simulink model "flightControlSystem"  (R2019b)
settings: Solver=ode3  StartTime=0  StopTime=TFinal  FixedStep=Ts  RelTol=1e-3  EnableMultiTasking=on
undefined symbols (not defined in the file): codertarget, Controller, DiscIntNeverNeededParam, Discrete, Estimator, g, init, Sensors, Time, Ts, Vehicle
libraries: simulink x35, vrlib x4, sharedtransform x3, ctrlSharedLib x2, sharedutil x1, parrotlib x1
(part 2 of 2)

== system flightControlSystem/Control System/Path Planning/Line Follower/Re-find track ==
  x_target : Inport  OutDataTypeStr=single
  y_target : Inport  Port=2  OutDataTypeStr=single
  x_cur : Inport  Port=3  OutDataTypeStr=single
  y_cur : Inport  Port=4  OutDataTypeStr=single
  MATLAB Function : MATLAB Function  TreatAsAtomicUnit=on
  Mux : Mux  Inputs=3
  Z_pos : Constant  Value=-1.1  OutDataTypeStr=single
  target_coordinates : Outport  OutDataTypeStr=single
  wires:
  Mux/1 -> target_coordinates/1
  Z_pos/1 -> Mux/3
  y_target/1 -> MATLAB Function/3(y_target)
  y_cur/1 -> MATLAB Function/4(y_cur)
  x_target/1 -> MATLAB Function/1(x_target)
  x_cur/1 -> MATLAB Function/2(x_cur)
  MATLAB Function/2(y) -> Mux/2
  MATLAB Function/1(x) -> Mux/1

== system flightControlSystem/Control System/State Estimator/Complementary Filter/If Action Subsystem ==
  rpy : Inport
  accel : Inport  Port=2
  Action Port : ActionPort  ActionPortLabel=if(u1 > 0)
  Demux : Demux  Outputs=3
  Demux1 : Demux  Outputs=3
  Divide : Product  Inputs=*/
  Gain : Gain  Gain=1-Estimator.gyroAngleUpdateAccWeight
  Gain1 : Gain  Gain=Estimator.gyroAngleUpdateAccWeight
  Gain2 : Gain  Gain=1/g
  Gain3 : Gain  Gain=Estimator.gyroAngleUpdateAccWeight
  Gain4 : Gain  Gain=1-Estimator.gyroAngleUpdateAccWeight
  Mux : Mux  Inputs=2
  Sum : Sum  Inputs=|++
  Sum1 : Sum  Inputs=|++
  Terminator1 : Terminator
  Trigonometric Function : Trigonometry  Operator=atan
  Trigonometric Function1 : Trigonometry  Operator=asin
  pitch,roll : Outport  VectorParamsAs1DForOutWhenUnconnected=off
  wires:
  accel/1 -> Demux/1
  Demux/2 -> Divide/1
  Demux/3 -> Divide/2
  Divide/1 -> Trigonometric Function/1
  Gain/1 -> Sum/1
  Trigonometric Function/1 -> Gain1/1
  Mux/1 -> pitch,roll/1
  Gain2/1 -> Trigonometric Function1/1
  Trigonometric Function1/1 -> Gain3/1
  Gain4/1 -> Sum1/1
  Gain3/1 -> Sum1/2
  Sum1/1 -> Mux/1
  Sum/1 -> Mux/2
  rpy/1 -> Demux1/1
  Demux1/1 -> Gain/1
  Demux1/2 -> Gain4/1
  Demux/1 -> Gain2/1
  Demux1/3 -> Terminator1/1
  Gain1/1 -> Sum/2

== system flightControlSystem/Control System/State Estimator/Complementary Filter/If Action Subsystem2 ==
  prin : Inport
  Action Port : ActionPort  ActionPortLabel=else
  prout : Outport  VectorParamsAs1DForOutWhenUnconnected=off
  wires:
  prin/1 -> prout/1

== system flightControlSystem/Control System/State Estimator/Complementary Filter/Wbe ==
  rpy : Inport  OutDataTypeStr=single
  Constant : Constant  Value=single(0)
  Create 3x3 Matrix : sharedutil/Create 3x3 Matrix  aMode=aMode
  Divide : Product  Inputs=*/
  Gain : Gain  Gain=-1
  Product{1..4} (4 alike) : Product
  Selector : Selector  InputPortWidth=3  IndexOptions=Index vector (dialog)  Indices=[1]  OutputSizes=1
  Selector1 : Selector  InputPortWidth=3  IndexOptions=Index vector (dialog)  Indices=[1]  OutputSizes=1
  Selector2 : Selector  InputPortWidth=3  IndexOptions=Index vector (dialog)  Indices=[2]  OutputSizes=1
  Selector3 : Selector  InputPortWidth=3  IndexOptions=Index vector (dialog)  Indices=[2]  OutputSizes=1
  Trigonometric Function : Trigonometry  Operator=sincos
  Wbe : Outport  VectorParamsAs1DForOutWhenUnconnected=off
  wires:
  Create 3x3 Matrix/1 -> Divide/1
  Product3/1 -> Create 3x3 Matrix/8
  Trigonometric Function/2 -> Selector1/1, Selector2/1
  Selector3/1 -> Product4/2, Product3/2
  Selector1/1 -> Product4/1, Product1/1, Create 3x3 Matrix/3
  Trigonometric Function/1 -> Selector3/1, Selector/1
  Product1/1 -> Create 3x3 Matrix/5
  Product2/1 -> Create 3x3 Matrix/6
  Selector2/1 -> Divide/2, Create 3x3 Matrix/7, Product2/1, Product1/2
  Gain/1 -> Product2/2
  Product4/1 -> Create 3x3 Matrix/9
  Constant/1 -> Create 3x3 Matrix/4, Create 3x3 Matrix/1
  Divide/1 -> Wbe/1
  rpy/1 -> Trigonometric Function/1
  Selector/1 -> Product3/1, Gain/1, Create 3x3 Matrix/2

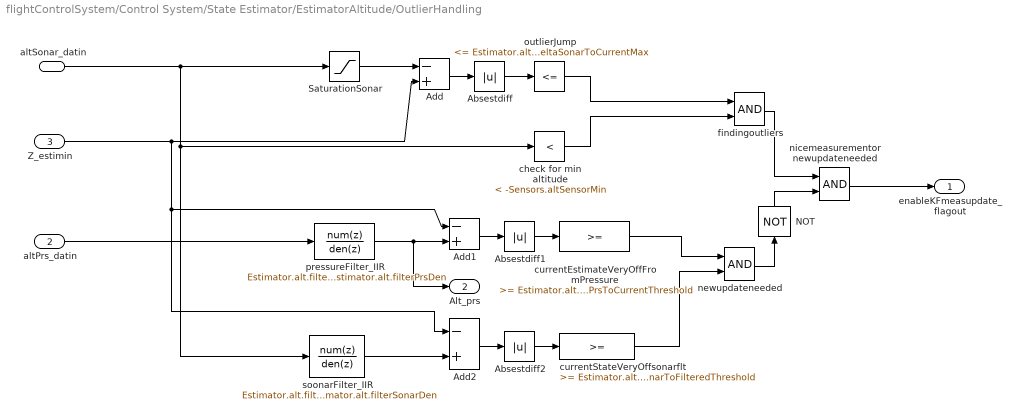
== system flightControlSystem/Control System/State Estimator/EstimatorAltitude/OutlierHandling ==
  altSonar_datin : Inport
  altPrs_datin : Inport  Port=2
  Z_estimin : Inport  Port=3
  Absestdiff : Abs
  Absestdiff1 : Abs
  Absestdiff2 : Abs
  Add : Sum  Inputs=-+
  Add1 : Sum  Inputs=-+
  Add2 : Sum  Inputs=-+
  NOT : Logic  Operator=NOT  IconShape=distinctive  AllPortsSameDT=off  OutDataTypeStr=boolean
  SaturationSonar : Saturate  UpperLimit=-Sensors.altSensorMin  LowerLimit=-inf
  check for min altitude : simulink/Logic and Bit Operations/Compare To Constant  relop=<  const=-Sensors.altSensorMin  OutDataTypeStr=boolean
  currentEstimateVeryOffFromPressure : simulink/Logic and Bit Operations/Compare To Constant  relop=>=  const=Estimator.alt.deltaPrsToCurrentThreshold  OutDataTypeStr=boolean
  currentStateVeryOffsonarflt : simulink/Logic and Bit Operations/Compare To Constant  relop=>=  const=Estimator.alt.deltaSonarToFilteredThreshold  OutDataTypeStr=boolean
  findingoutliers : Logic  AllPortsSameDT=off  OutDataTypeStr=boolean
  newupdateneeded : Logic  AllPortsSameDT=off  OutDataTypeStr=boolean
  nicemeasurementor newupdateneeded : Logic  AllPortsSameDT=off  OutDataTypeStr=boolean
  outlierJump : simulink/Logic and Bit Operations/Compare To Constant  relop=<=  const=Estimator.alt.deltaSonarToCurrentMax  OutDataTypeStr=boolean
  pressureFilter_IIR : DiscreteFilter  Numerator=Estimator.alt.filterPrsNum  Denominator=Estimator.alt.filterPrsDen
  soonarFilter_IIR : DiscreteFilter  Numerator=Estimator.alt.filterSonarNum  Denominator=Estimator.alt.filterSonarDen
  enableKFmeasupdate_flagout : Outport  VectorParamsAs1DForOutWhenUnconnected=off
  Alt_prs : Outport  Port=2  VectorParamsAs1DForOutWhenUnconnected=off
  wires:
  Add1/1 -> Absestdiff1/1
  nicemeasurementor newupdateneeded/1 -> enableKFmeasupdate_flagout/1
  findingoutliers/1 -> nicemeasurementor newupdateneeded/1
  check for min altitude/1 -> findingoutliers/2
  outlierJump/1 -> findingoutliers/1
  SaturationSonar/1 -> Add/1
  Absestdiff/1 -> outlierJump/1
  Add/1 -> Absestdiff/1
  newupdateneeded/1 -> NOT/1
  Absestdiff2/1 -> currentStateVeryOffsonarflt/1
  altSonar_datin/1 -> SaturationSonar/1, soonarFilter_IIR/1, check for min altitude/1
  currentEstimateVeryOffFromPressure/1 -> newupdateneeded/1
  Z_estimin/1 -> Add1/1, Add2/1, Add/2
  Add2/1 -> Absestdiff2/1
  currentStateVeryOffsonarflt/1 -> newupdateneeded/2
  pressureFilter_IIR/1 -> Alt_prs/1, Add1/2
  altPrs_datin/1 -> pressureFilter_IIR/1
  soonarFilter_IIR/1 -> Add2/2
  Absestdiff1/1 -> currentEstimateVeryOffFromPressure/1
  NOT/1 -> nicemeasurementor newupdateneeded/2

== system flightControlSystem/Control System/State Estimator/EstimatorXYPosition/EstimatorVelocity ==
  opticalFlow_datin : Inport
  Z_estimin : Inport  Port=2  SampleTime=Ts
  sensorIMU_datin : Inport  Port=3
  orient_estimin : Inport  Port=4
  " " : Product  Inputs=**
  AccelerationHandling : Subsystem
  Compare To Constant : simulink/Logic and Bit Operations/Compare To Constant  relop=<  const=200*4  OutDataTypeStr=boolean
  Counter Free-Running : simulink/Sources/Counter Free-Running  NumBits=32  tsamp=-1
  DataHandling : Subsystem
  Delay : Delay  DelayLength=1  InitialCondition=0
  Gain : Gain  Gain=-1
  KalmanFilter_dxdy : ctrlSharedLib/Kalman Filter  TimeDomain=Discrete-Time  UseCurrentEstimator=on  ModelSource=Individual A, B, C, D matrices  ModelSourceVariable=ss(0.95,1,1,0,1)  A=eye(2)  B=Ts*eye(2)  C=eye(2)  D=0  NumberOfStates=1  NumberOfInputs=1  NumberOfOutputs=1  InitialEstimateSource=Dialog  X0=0  P0=10  UseK=off  UseGH=on  NumberOfProcessNoiseInputs=1  G=Estimator.pos.kfVelo.G  TimeInvariantG=on  H=Estimator.pos.kfVelo.H  TimeInvariantH=on  Q=Estimator.pos.kfVelo.Q  TimeInvariantQ=on  R=Estimator.pos.kfVelo.R  TimeInvariantR=on  N=Estimator.pos.kfVelo.N  TimeInvariantN=on  AddInputPort=on  AddEnablePort=on  OutputEstimatedY=off  OutputP=off  Ts=-1
      settings: SourceProductBaseCode=CT
  Select dxy : Selector  InputPortWidth=3  IndexOptions=Index vector (dialog)  Indices=[1 2]  OutputSizes=1
  Switch : Switch  Criteria=u2 > Threshold
  Z_estimin1 : InportShadow  Port=2  SampleTime=Ts
  opticalFlowErrorCorrect : Gain  Gain=1.15
  dxy_estimout : Outport  VectorParamsAs1DForOutWhenUnconnected=off
  wires:
  Delay/1 -> DataHandling/5(dxyOF_datin)
  Z_estimin/1 -> DataHandling/1(Z_estimin), AccelerationHandling/4(Z_estimin)
  KalmanFilter_dxdy/1 -> dxy_estimout/1, Delay/1
  sensorIMU_datin/1 -> AccelerationHandling/2(sensorIMU_datin), DataHandling/3(sensorIMU_datin)
  orient_estimin/1 -> AccelerationHandling/3(orient_estimin), DataHandling/2(orient_estimin)
  Select dxy/1 -> KalmanFilter_dxdy/2, AccelerationHandling/1(dxy_estimin), DataHandling/4(dxy_estimin)
  AccelerationHandling/1(acceleration_world) -> KalmanFilter_dxdy/1
  DataHandling/1(enable_flag) -> KalmanFilter_dxdy/3
  Switch/1 -> Select dxy/1
  " "/1 -> opticalFlowErrorCorrect/1
  Gain/1 -> " "/2
  opticalFlowErrorCorrect/1 -> Switch/3
  Compare To Constant/1 -> Switch/2
  opticalFlow_datin/1 -> " "/1, Switch/1
  Z_estimin1/1 -> Gain/1
  Counter Free-Running/1 -> Compare To Constant/1

== system flightControlSystem/Control System/State Estimator/EstimatorXYPosition/EstimatorXYPosition ==
  note: Switching from orientationControl to Position
      | control reset the current world position estimate
      | (happens when using no markers)
  dxy_estimin : Inport
  orient_estimin : Inport  Port=2  SampleTime=Ts
  controlModePosVSOrient_flagin : Inport  Port=3
  dz_estimin : Inport  Port=4
  Math Function : Math  Operator=transpose  SaturateOnIntegerOverflow=on
  Mux2 : Mux  Inputs=2
  Product : Product  Multiplication=Matrix(*)
  Rotation Angles to Direction Cosine Matrix : sharedtransform/Rotation Angles to Direction Cosine Matrix  rotationOrder=ZYX  aMode=aMode
      settings: SourceProductBaseCode=AE
  SelectdXY : Selector  InputPortWidth=3  IndexOptions=Index vector (dialog)  Indices=[1 2]  OutputSizes=1
  SimplyIntegrateVelocity : DiscreteIntegrator  ExternalReset=rising  SampleTime=Ts  ICPrevOutput=DiscIntNeverNeededParam  ICPrevScaledInput=DiscIntNeverNeededParam
  XY_estimout : Outport  VectorParamsAs1DForOutWhenUnconnected=off
  wires:
  controlModePosVSOrient_flagin/1 -> SimplyIntegrateVelocity/2
  Product/1 -> SelectdXY/1
  Mux2/1 -> Product/2
  dz_estimin/1 -> Mux2/2
  SimplyIntegrateVelocity/1 -> XY_estimout/1
  dxy_estimin/1 -> Mux2/1
  orient_estimin/1 -> Rotation Angles to Direction Cosine Matrix/1
  Rotation Angles to Direction Cosine Matrix/1 -> Math Function/1
  SelectdXY/1 -> SimplyIntegrateVelocity/1
  Math Function/1 -> Product/1

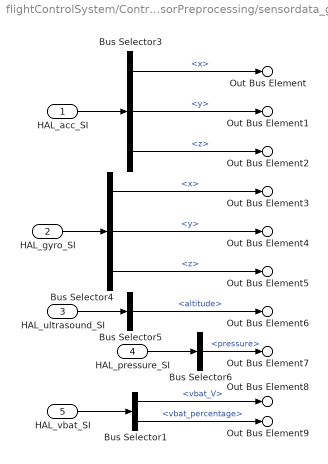
== system flightControlSystem/Control System/State Estimator/SensorPreprocessing/sensordata_group ==
  HAL_acc_SI : Inport  OutDataTypeStr=Bus: HAL_acc_SI_t
  HAL_gyro_SI : Inport  Port=2  OutDataTypeStr=Bus: HAL_gyro_SI_t
  HAL_ultrasound_SI : Inport  Port=3  OutDataTypeStr=Bus: HAL_ultrasound_SI_t
  HAL_pressure_SI : Inport  Port=4  OutDataTypeStr=Bus: HAL_pressure_SI_t
  HAL_vbat_SI : Inport  Port=5  OutDataTypeStr=Bus: HAL_vbat_SI_t
  Bus Selector1 : BusSelector  OutputSignals=vbat_V,vbat_percentage
  Bus Selector3 : BusSelector  OutputSignals=x,y,z
  Bus Selector4 : BusSelector  OutputSignals=x,y,z
  Bus Selector5 : BusSelector  OutputSignals=altitude
  Bus Selector6 : BusSelector  OutputSignals=pressure
  Out Bus Element : Outport  VectorParamsAs1DForOutWhenUnconnected=off  PortName=sensordata_datin  Element=ddx
  Out Bus Element1 : Outport  VectorParamsAs1DForOutWhenUnconnected=off  PortName=sensordata_datin  Element=ddy
  Out Bus Element2 : Outport  VectorParamsAs1DForOutWhenUnconnected=off  PortName=sensordata_datin  Element=ddz
  Out Bus Element3 : Outport  VectorParamsAs1DForOutWhenUnconnected=off  PortName=sensordata_datin  Element=p
  Out Bus Element4 : Outport  VectorParamsAs1DForOutWhenUnconnected=off  PortName=sensordata_datin  Element=q
  Out Bus Element5 : Outport  VectorParamsAs1DForOutWhenUnconnected=off  PortName=sensordata_datin  Element=r
  Out Bus Element6 : Outport  VectorParamsAs1DForOutWhenUnconnected=off  PortName=sensordata_datin  Element=altitude_sonar
  Out Bus Element7 : Outport  VectorParamsAs1DForOutWhenUnconnected=off  PortName=sensordata_datin  Element=prs
  Out Bus Element8 : Outport  VectorParamsAs1DForOutWhenUnconnected=off  PortName=sensordata_datin  Element=vbat_V
  Out Bus Element9 : Outport  VectorParamsAs1DForOutWhenUnconnected=off  PortName=sensordata_datin  Element=vbat_percentage
  wires:
  HAL_gyro_SI/1 -> Bus Selector4/1
  HAL_acc_SI/1 -> Bus Selector3/1
  HAL_pressure_SI/1 -> Bus Selector6/1
  HAL_ultrasound_SI/1 -> Bus Selector5/1
  Bus Selector4/1 -> Out Bus Element3/1  "<x>"
  Bus Selector3/3 -> Out Bus Element2/1  "<z>"
  Bus Selector4/3 -> Out Bus Element5/1  "<z>"
  Bus Selector5/1 -> Out Bus Element6/1  "<altitude>"
  Bus Selector6/1 -> Out Bus Element7/1  "<pressure>"
  Bus Selector4/2 -> Out Bus Element4/1  "<y>"
  Bus Selector3/1 -> Out Bus Element/1  "<x>"
  Bus Selector3/2 -> Out Bus Element1/1  "<y>"
  Bus Selector1/1 -> Out Bus Element8/1  "<vbat_V>"
  HAL_vbat_SI/1 -> Bus Selector1/1
  Bus Selector1/2 -> Out Bus Element9/1  "<vbat_percentage>"

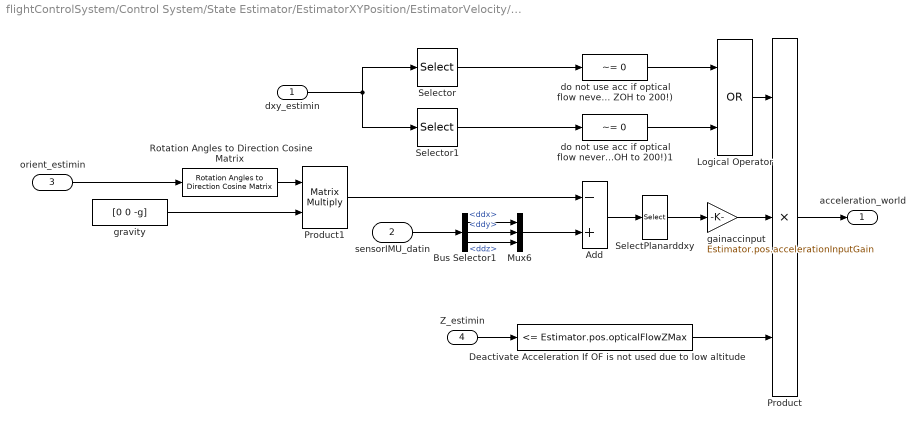
== system flightControlSystem/Control System/State Estimator/EstimatorXYPosition/EstimatorVelocity/AccelerationHandling ==
  dxy_estimin : Inport
  sensorIMU_datin : Inport  Port=2
  orient_estimin : Inport  Port=3
  Z_estimin : Inport  Port=4
  Add : Sum  Inputs=-+
  Bus Selector1 : BusSelector  OutputSignals=ddx,ddy,ddz
  Deactivate Acceleration If OF is not used due to low altitude : simulink/Logic and Bit Operations/Compare To Constant  relop=<=  const=Estimator.pos.opticalFlowZMax  OutDataTypeStr=boolean
  Logical Operator : Logic  Operator=OR  AllPortsSameDT=off  OutDataTypeStr=boolean
  Mux6 : Mux  Inputs=3
  Product : Product  Inputs=3
  Product1 : Product  Multiplication=Matrix(*)
  Rotation Angles to Direction Cosine Matrix : sharedtransform/Rotation Angles to Direction Cosine Matrix  rotationOrder=ZYX  aMode=aMode
      settings: SourceProductBaseCode=AE
  SelectPlanarddxy : Selector  InputPortWidth=3  IndexOptions=Index vector (dialog)  Indices=[1 2]  OutputSizes=1
  Selector : Selector  InputPortWidth=2  IndexOptions=Index vector (dialog)  Indices=1  OutputSizes=1
  Selector1 : Selector  InputPortWidth=2  IndexOptions=Index vector (dialog)  Indices=2  OutputSizes=1
  do not use acc if optical flow never available (Note OF@60Hz but ZOH to 200!) : simulink/Logic and Bit Operations/Compare To Constant  relop=~=  const=0  OutDataTypeStr=boolean
  do not use acc if optical flow never available (Note OF@60Hz but ZOH to 200!)1 : simulink/Logic and Bit Operations/Compare To Constant  relop=~=  const=0  OutDataTypeStr=boolean
  gainaccinput : Gain  Gain=Estimator.pos.accelerationInputGain  OutDataTypeStr=single
  gravity : Constant  Value=[0 0 -g]
  acceleration_world : Outport  OutDataTypeStr=single  VectorParamsAs1DForOutWhenUnconnected=off
  wires:
  do not use acc if optical flow never available (Note OF@60Hz but ZOH to 200!)1/1 -> Logical Operator/2
  do not use acc if optical flow never available (Note OF@60Hz but ZOH to 200!)/1 -> Logical Operator/1
  Logical Operator/1 -> Product/1
  Selector1/1 -> do not use acc if optical flow never available (Note OF@60Hz but ZOH to 200!)1/1
  Selector/1 -> do not use acc if optical flow never available (Note OF@60Hz but ZOH to 200!)/1
  dxy_estimin/1 -> Selector1/1, Selector/1
  Product/1 -> acceleration_world/1
  Deactivate Acceleration If OF is not used due to low altitude/1 -> Product/3
  Z_estimin/1 -> Deactivate Acceleration If OF is not used due to low altitude/1
  Add/1 -> SelectPlanarddxy/1
  Product1/1 -> Add/1
  gravity/1 -> Product1/2
  gainaccinput/1 -> Product/2
  SelectPlanarddxy/1 -> gainaccinput/1
  Bus Selector1/3 -> Mux6/3  "<ddz>"
  Bus Selector1/1 -> Mux6/1  "<ddx>"
  sensorIMU_datin/1 -> Bus Selector1/1
  Mux6/1 -> Add/2
  Bus Selector1/2 -> Mux6/2  "<ddy>"
  orient_estimin/1 -> Rotation Angles to Direction Cosine Matrix/1
  Rotation Angles to Direction Cosine Matrix/1 -> Product1/1

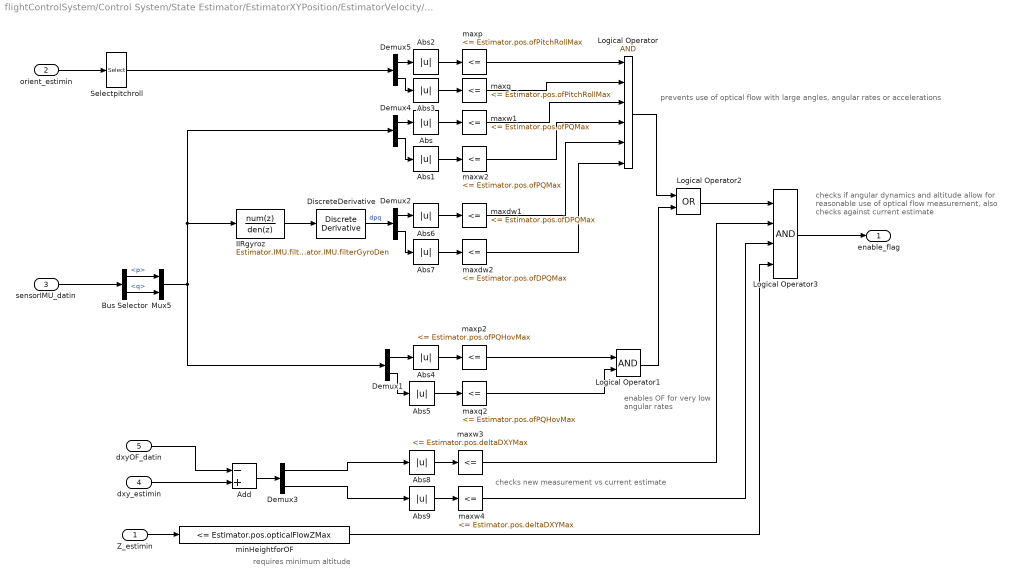
== system flightControlSystem/Control System/State Estimator/EstimatorXYPosition/EstimatorVelocity/DataHandling ==
  note: prevents use of optical flow with large angles, angular rates or accelerations
  note: enables OF for very
      | low angular rates
  note: checks if angular dynamics and altitude allow for
      | reasonable use of optical flow measurement,
      | also checks against current estimate
  note: checks new measurement vs current estimate
  note: requires minimum altitude
  Z_estimin : Inport
  orient_estimin : Inport  Port=2
  sensorIMU_datin : Inport  Port=3
  dxy_estimin : Inport  Port=4
  dxyOF_datin : Inport  Port=5
  Abs{,1..9} (10 alike) : Abs
  Add : Sum  Inputs=-+
  Bus Selector : BusSelector  OutputSignals=p,q
  Demux{1..5} (5 alike) : Demux  Outputs=2
  DiscreteDerivative : simulink/Discrete/Discrete Derivative  gainval=1.0  ICPrevScaledInput=0.0  OutMin=[]  OutMax=[]  OutDataType=fixdt(1, 16)  OutScaling=2^-10  DoSatur=off
  IIRgyroz : DiscreteFilter  Numerator=Estimator.IMU.filterGyroNum  Denominator=Estimator.IMU.filterGyroDen
  Logical Operator : Logic  Inputs=6  AllPortsSameDT=off  OutDataTypeStr=boolean
  Logical Operator1 : Logic  AllPortsSameDT=off  OutDataTypeStr=boolean
  Logical Operator2 : Logic  Operator=OR  AllPortsSameDT=off  OutDataTypeStr=boolean
  Logical Operator3 : Logic  Inputs=4  AllPortsSameDT=off  OutDataTypeStr=boolean
  Mux5 : Mux  Inputs=2
  Selectpitchroll : Selector  InputPortWidth=3  IndexOptions=Index vector (dialog)  Indices=[2 3]  OutputSizes=1
  maxdw1 : simulink/Logic and Bit Operations/Compare To Constant  relop=<=  const=Estimator.pos.ofDPQMax  OutDataTypeStr=boolean
  maxdw2 : simulink/Logic and Bit Operations/Compare To Constant  relop=<=  const=Estimator.pos.ofDPQMax  OutDataTypeStr=boolean
  maxp : simulink/Logic and Bit Operations/Compare To Constant  relop=<=  const=Estimator.pos.ofPitchRollMax  OutDataTypeStr=boolean
  maxp2 : simulink/Logic and Bit Operations/Compare To Constant  relop=<=  const=Estimator.pos.ofPQHovMax  OutDataTypeStr=boolean
  maxq : simulink/Logic and Bit Operations/Compare To Constant  relop=<=  const=Estimator.pos.ofPitchRollMax  OutDataTypeStr=boolean
  maxq2 : simulink/Logic and Bit Operations/Compare To Constant  relop=<=  const=Estimator.pos.ofPQHovMax  OutDataTypeStr=boolean
  maxw1 : simulink/Logic and Bit Operations/Compare To Constant  relop=<=  const=Estimator.pos.ofPQMax  OutDataTypeStr=boolean
  maxw2 : simulink/Logic and Bit Operations/Compare To Constant  relop=<=  const=Estimator.pos.ofPQMax  OutDataTypeStr=boolean
  maxw3 : simulink/Logic and Bit Operations/Compare To Constant  relop=<=  const=Estimator.pos.deltaDXYMax  OutDataTypeStr=boolean
  maxw4 : simulink/Logic and Bit Operations/Compare To Constant  relop=<=  const=Estimator.pos.deltaDXYMax  OutDataTypeStr=boolean
  minHeightforOF : simulink/Logic and Bit Operations/Compare To Constant  relop=<=  const=Estimator.pos.opticalFlowZMax  OutDataTypeStr=boolean
  enable_flag : Outport  VectorParamsAs1DForOutWhenUnconnected=off
  wires:
  minHeightforOF/1 -> Logical Operator3/4
  IIRgyroz/1 -> DiscreteDerivative/1
  Mux5/1 -> Demux1/1, IIRgyroz/1, Demux4/1
  maxw4/1 -> Logical Operator3/3
  maxw3/1 -> Logical Operator3/2
  dxyOF_datin/1 -> Add/1
  Demux3/2 -> Abs9/1
  Demux3/1 -> Abs8/1
  dxy_estimin/1 -> Add/2
  Add/1 -> Demux3/1
  Abs9/1 -> maxw4/1
  Abs8/1 -> maxw3/1
  Logical Operator2/1 -> Logical Operator3/1
  Logical Operator3/1 -> enable_flag/1
  DiscreteDerivative/1 -> Demux2/1  "dpq"
  Demux2/2 -> Abs7/1
  Demux2/1 -> Abs6/1
  Abs7/1 -> maxdw2/1
  Abs6/1 -> maxdw1/1
  Logical Operator1/1 -> Logical Operator2/2
  Demux1/2 -> Abs5/1
  Demux1/1 -> Abs4/1
  Abs5/1 -> maxq2/1
  Abs4/1 -> maxp2/1
  Abs3/1 -> maxq/1
  Abs2/1 -> maxp/1
  Demux4/2 -> Abs1/1
  Demux4/1 -> Abs/1
  Abs1/1 -> maxw2/1
  Abs/1 -> maxw1/1
  Z_estimin/1 -> minHeightforOF/1
  Logical Operator/1 -> Logical Operator2/1
  maxw1/1 -> Logical Operator/3
  Bus Selector/1 -> Mux5/1  "<p>"
  Selectpitchroll/1 -> Demux5/1
  sensorIMU_datin/1 -> Bus Selector/1
  maxq2/1 -> Logical Operator1/2
  Bus Selector/2 -> Mux5/2  "<q>"
  maxp/1 -> Logical Operator/1
  maxw2/1 -> Logical Operator/4
  orient_estimin/1 -> Selectpitchroll/1
  maxdw1/1 -> Logical Operator/5
  maxdw2/1 -> Logical Operator/6
  maxq/1 -> Logical Operator/2
  Demux5/1 -> Abs2/1
  Demux5/2 -> Abs3/1
  maxp2/1 -> Logical Operator1/1

== matlab function flightControlSystem/Image Processing System/Circle Finder ==
  data: BW input; circleFound output; coordinates output
function [circleFound, coordinates] = FindTheCircle(BW)

red = 0;

circleFound = false;
coordinates = [0,0];
row = 120;
col = 160;

%%%%NEEDS FOCUS
diameter = 37;
margin = 1; 

%stepsize = 1; %e.g. could change to 2 to check every 2nd column
for i = 1:1:col %traverse columns in BW image
    red_px_count = 0; %count of consecutive red pixels in a column - is updated as we traverse columns
    for j = 1:1:(row - 1) %traverse rows in column - not to last row element
        %Adjusting red_px_count 
        if (BW(j,i) == red) %i.e. if pixel is red
            red_px_count = red_px_count + 1;
        else 
            red_px_count = 0;
        end
        
        if ( (red_px_count <= diameter + margin) && (red_px_count >= diameter - margin) && (BW(j+1,i) ~= red))
            %centre row is around/at (j - (red_px_count-1)/2) depending on
            %whether result is a decimal or integer
            row_pos = (j - (red_px_count-1)/2);
            if( horizontal_test(floor(row_pos),i,BW) == true )
                circleFound = true;
                coordinates = [i,floor(row_pos)]; %returning col,row format as thats what is currently expected at path planning
                break;
            elseif (horizontal_test(ceil(row_pos),i,BW) == true )
                circleFound = true;
                coordinates = [i, ceil(row_pos)]; %col, row format
                break;
            end
        end
    end
end

function circleFound = horizontal_test(row,col,BW)

red = 0;

num_col = 160;
circleFound = false;

diameter = 37;
diameter_margin = 1;

centre_margin = 1;
red_px_count = 0; %count of consecutive red pixels in a column - is updated as we traverse columns

for i = 1:1:(num_col-1) %traverse columns in BW image
        %Adjusting red_px_count
        if (BW(row,i) == red) %i.e. if pixel is red
            red_px_count = red_px_count + 1;
        else
            red_px_count = 0;
        end
        %Checking if red_px_count = ~ diameter of circle
        if ( (red_px_count <= diameter + diameter_margin) && (red_px_count >= diameter - diameter_margin) && BW(row,i+1) ~= red )
            col_no = i - (red_px_count - 1)/2;
            if ( col_no <= col + centre_margin && col_no >= col - centre_margin )
                circleFound = true;
                break;
            end
        end
end

== matlab function flightControlSystem/Image Processing System/MATLAB Function1 ==
  data: r input; r1 output; g input; b input; av_points input; g1 output; b1 output
%FUNCTION DESCRIPTION

% the values for r1,g1,b1 which we pass out are the same as r,g,b inputs
% except r1,g1,b1 values are changed to highlight: 
%
% - origin/centre of image
% 
% - gridlines used in 'Waypoint Finder' block
% 
% - 4 average points along 4 gridlines used to calculate unit vectors in
%  'Waypoint Finder' block

function [r1,g1,b1] = fcn(r,g,b,av_points)
% setting values for r1,g1,b1 equal to r,g,b inputs
r1=r;
g1=g;
b1=b;

% highlighting origin (centre of image) black (black's r,g,b value is 1,1,1)
r1(60,80) = 1;
g1(60,80) = 1;
b1(60,80) = 1;


% highlighting gridlines used in 'Waypoint Finder' block black
% (black's r,g,b value is 1,1,1)
% gridline 1
r1(40,:) = 1;
g1(40,:) = 1;
b1(40,:) = 1;

% gridline 2
r1(80,:) = 1;
g1(80,:) = 1;
b1(80,:) = 1;

% gridline 3
r1(:,60) = 1;
g1(:,60) = 1;
b1(:,60) = 1;

% gridline 4
r1(:,100) = 1;
g1(:,100) = 1;
b1(:,100) = 1;

% highlighting av_points white if valid points are received hence isnan
%(white's r,g,b value is 255,255,255)

% point 1
if ~isnan(av_points(1:2))
r1(av_points(1),av_points(2)) = 255;
g1(av_points(1),av_points(2)) = 255;
b1(av_points(1),av_points(2)) = 255;
end

% point 2
if ~isnan(av_points(3:4))
r1(av_points(3),av_points(4)) = 255;
g1(av_points(3),av_points(4)) = 255;
b1(av_points(3),av_points(4)) = 255;
end

% point 3
if ~isnan(av_points(5:6))
r1(av_points(5),av_points(6)) = 255;
g1(av_points(5),av_points(6)) = 255;
b1(av_points(5),av_points(6)) = 255;
end

% point 4
if ~isnan(av_points(7:8))
r1(av_points(7),av_points(8)) = 255;
g1(av_points(7),av_points(8)) = 255;
b1(av_points(7),av_points(8)) = 255;
end

== matlab function flightControlSystem/Image Processing System/rgb to boolean ==
  data: r input; BW output; g input; b input
function BW = fcn(r, g, b)
%Threshold values for r,g,b components
Th_r = 190;
Th_g = 90;
Th_b = 90;

BW = ~( r > Th_r & g < Th_g & b < Th_b);

== matlab function flightControlSystem/Control System/Path Planning/Go to centre/Coord to Vector ==
  data: coord input; x_vec output; y_vec output; z_vec output; over_centre output; yaw input; pitch input; roll input
function [x_vec, y_vec, z_vec, over_centre] = fcn(coord,yaw,pitch,roll)
%This function will take the coordinates of the target circle with the top
%left pixel as the origin and convert it to a vector with the origin as the
%centre of the image.
%It then tells the drone to land at it's centre

%Input: coord, coordinates of target circle
%Output: vec2target, vector to center pointing from center of image
%       x_vec, x component of vector to fly to
%       y_vec, same as for x_vec
%       z_vec, same as for x_vec
%       over_centre, flag for when over circle
    %radius = 19;
    threshold = 10;
    %Convert coordinate space to origin at centre
    coord = coord - [80, 60]; %Pixel positions with centre as origin
    vec2target = coord.*[1, -1];
    
    nrm = norm(vec2target);
    x_vec = vec2target(2)/nrm;
    y_vec = vec2target(1)/nrm;
    z_vec = -1.1;
    over_centre = false;
    
    %Tell drone to land if above the circle
    if ( nrm < threshold & yaw < 0.0001 & pitch < 0.0001 & roll < 0.0001 )
        x_vec = 0;
        y_vec = 0;
        over_centre = true;
    end

== stateflow chart flightControlSystem/Control System/Path Planning/Line Follower/State Machine ==
  state Lost
    entry:
    mode = 1;
    last_valid_vec = [(xp - xp_min1) (yp - yp_min1)];
    x_target = (xp+xp_min1)/2;
    y_target = (yp+yp_min1)/2;
  state NormalOp
    entry:
    mode = 0;
    during:
    last_valid_vec = [(xcur - xcur_minus1) (ycur - ycur_minus1)];
  (default) -> NormalOp
  NormalOp -> Lost : [lost]
  Lost -> NormalOp : [~lost & abs(xcur-x_target) < closeness_margin & abs(ycur-y_target) < closeness_margin]
  data: lost input; mode output; xcur input; xcur_minus1 input; ycur input; ycur_minus1 input; last_valid_vec output; closeness_margin constant double =0.005; x_target output single; y_target output single; xp input; xp_min1 input; yp input; yp_min1 input

== matlab function flightControlSystem/Control System/Path Planning/Line Follower/MATLAB Function ==
  data: vecs input; lost output
function lost  = fcn(vecs)
vecs_nan = isnan(vecs);
if( (vecs_nan(1) || vecs_nan(2)) && (vecs_nan(3) || vecs_nan(4)) && (vecs_nan(5) || vecs_nan(6)) && (vecs_nan(7) || vecs_nan(8)) )
    lost = true;
else
    lost = false;
end

== matlab function flightControlSystem/Control System/Path Planning/Line Follower/Normal Operation/Best Path ==
  data: vecs input; x_best output; last_travelled_vec input; y_best output
%vecs = [y1, x1, y2, x2, y3, x3, y4, x4]
%-> array containing up to 4 valid unit vectors
 
%We will choose the unit vector from vecs which is most similar to the 
%unit vector we travelled (in the direction of) in the previous time step
 
%i.e. We choose the vector from vecs which gives the largest value 
%from this eq.
%(x_p + vecs[xi])^2 + (y_p + vecs[yi]))^2 
 
%e.g. if one vector told us to go back relative to direction we were 
%just travelling, it's x and y components would cancel with the x and 
%y components of the vector we last travelled through and we would discount
%it as a valid vector to follow
 
function [x_best,y_best] = best_vector(vecs,last_travelled_vec)
    x_p = last_travelled_vec(1);
    y_p = last_travelled_vec(2);
    
    %initialising variables
    Biggest_sum = single(0);
    sum = single(0);
    n_best = 0; %used to mark index of best vector in vecs
   
    %iterate through vecs
    for n = 0:3
        %Finding vector in vecs most in line with previous direction travelled 
        sum = (x_p + vecs(2+2*n))^2 + (y_p + vecs(1+2*n))^2;
        if sum > Biggest_sum
            Biggest_sum = sum;
            n_best = n;
        end
    end
        x_best = vecs(2+2*n_best);
        y_best = vecs(1+2*n_best);

end

== stateflow chart flightControlSystem/Control System/Path Planning/State Machine ==
  state Takeoff
    entry:
    curr_state = 1;
  state LineFollower
    entry:
    curr_state = 2;
  note: Wait till flight altitude reached
  state Circle_Found
    entry:
    curr_state = 3;
  state Land
    entry:
    curr_state = 4;
  (default) -> Takeoff
  Takeoff -> LineFollower : [Z<-1.09]
  LineFollower -> Circle_Found : [circle_found]
  Circle_Found -> Land : [over_centre]
  data: circle_found input; Z input; over_centre input; curr_state output

== matlab function flightControlSystem/Image Processing System/Waypoint Finder1/Find X_Waypoints ==
  data: BW input; Waypoint output; row input; av_point output
% Function to find the average y position of red pixels along a given row
%
% NB!!!!
% The y-axis as we refer to it in this project runs horizontally, 
% parallel to rows, like a traditional x-axis would
%
% The x-axis runs parallel to columns, like a traditional y-axis would

function [Waypoint,av_point] = Find_X_Waypoints(BW, row)

dimensions = size(BW);
width = dimensions(2); % Number of horizontal pixels (i.e. num of cols)

Sum_pxPos = 0;  % Running sum of y-positions of red pixels
num_red = 0;    % Running sum of red pixels found

for i = 1:width % iterate across colums in specific row
    if(BW(row, i) == false) % i.e. we have found a red pixel ...
        Sum_pxPos = Sum_pxPos + i;
        num_red = num_red + 1;
    end
end

% Average position of red pixels in row (specific row passed into this fn)
avg_px_position = Sum_pxPos/num_red;

% location in row,col format of average red pixel location in specific row
% used for debugging
av_point = [row,round(avg_px_position)];

% change this format!!!!
Waypoint = [avg_px_position, row];  % Pixel positions with bottom left as origin
Waypoint = Waypoint - [80, 60];     % Pixel positions with centre as origin
Waypoint = Waypoint.*[1, -1];

== matlab function flightControlSystem/Image Processing System/Waypoint Finder1/Find X_Waypoints1 ==
  data: BW input; Waypoint output; row input; av_point output
% Function to find the average y position of red pixels along a given row
%
% NB!!!!
% The y-axis as we refer to it in this project runs horizontally, 
% parallel to rows, like a traditional x-axis would
%
% The x-axis runs parallel to columns, like a traditional y-axis would

function [Waypoint,av_point] = Find_X_Waypoints(BW, row)

dimensions = size(BW);
width = dimensions(2); % Number of horizontal pixels (i.e. num of cols)

Sum_pxPos = 0;  % Running sum of y-positions of red pixels
num_red = 0;    % Running sum of red pixels found

for i = 1:width % iterate across colums in specific row
    if(BW(row, i) == false) % i.e. we have found a red pixel ...
        Sum_pxPos = Sum_pxPos + i;
        num_red = num_red + 1;
    end
end

% Average position of red pixels in row (specific row passed into this fn)
avg_px_position = Sum_pxPos/num_red;

% location in row,col format of average red pixel location in specific row
% used for debugging
av_point = [row,round(avg_px_position)];

% change this format!!!!
Waypoint = [avg_px_position, row];  % Pixel positions with bottom left as origin
Waypoint = Waypoint - [80, 60];     % Pixel positions with centre as origin
Waypoint = Waypoint.*[1, -1];

== matlab function flightControlSystem/Image Processing System/Waypoint Finder1/Find Y_Waypoint ==
  data: BW input; Waypoint output; col input; av_point output
% Function to find the average x position of red pixels for a given column
%
% NB!!!!
% The y-axis as we refer to it in this project runs horizontally, 
% parallel to rows, like a traditional x-axis would
%
% The x-axis runs parallel to columns, like a traditional y-axis would

function [Waypoint,av_point] = Find_Y_Waypoints(BW, col)

dimensions = size(BW);
height = dimensions(1); % Number of vertical pixels (i.e. num rows)

Sum_pxPos = 0;  % Running sum of x-positions of red pixels
num_red = 0;    % Running sum of red pixels found

for i = 1:height% iterate across rows in specific col
    if(BW(i,col) == false) % i.e. we have found a red pixel ...
        Sum_pxPos = Sum_pxPos + i;
        num_red = num_red + 1;
    end
end

% Average position of red pixels in col (specific col passed into this fn)
avg_px_position = Sum_pxPos/num_red;

% location in row,col format of average red pixel location in specific row
% used for debugging
av_point = [round(avg_px_position),col];

% change this format!!!!
Waypoint = [col, avg_px_position];  %Pixel positions with bottom left as origin
Waypoint = Waypoint - [80, 60];     %Pixel positions with centre as origin
Waypoint = Waypoint.*[1, -1];

== matlab function flightControlSystem/Image Processing System/Waypoint Finder1/Find Y_Waypoint1 ==
  data: BW input; Waypoint output; col input; av_point output
% Function to find the average x position of red pixels for a given column
%
% NB!!!!
% The y-axis as we refer to it in this project runs horizontally, 
% parallel to rows, like a traditional x-axis would
%
% The x-axis runs parallel to columns, like a traditional y-axis would

function [Waypoint,av_point] = Find_Y_Waypoints(BW, col)

dimensions = size(BW);
height = dimensions(1); % Number of vertical pixels (i.e. num rows)

Sum_pxPos = 0;  % Running sum of x-positions of red pixels
num_red = 0;    % Running sum of red pixels found

for i = 1:height% iterate across rows in specific col
    if(BW(i,col) == false) % i.e. we have found a red pixel ...
        Sum_pxPos = Sum_pxPos + i;
        num_red = num_red + 1;
    end
end

% Average position of red pixels in col (specific col passed into this fn)
avg_px_position = Sum_pxPos/num_red;

% location in row,col format of average red pixel location in specific row
% used for debugging
av_point = [round(avg_px_position),col];

% change this format!!!!
Waypoint = [col, avg_px_position];  %Pixel positions with bottom left as origin
Waypoint = Waypoint - [80, 60];     %Pixel positions with centre as origin
Waypoint = Waypoint.*[1, -1];

== matlab function flightControlSystem/Control System/Path Planning/Line Follower/Re-find track/MATLAB Function ==
  data: x output; x_target input; y output; x_cur input; y_target input; y_cur input
function [x,y] = fcn(x_target,x_cur,y_target,y_cur)
x = (x_target+x_cur)/2;
y = (y_target+y_cur)/2;
